simulink model "Curvature_lookup_table"  (R2021a)
settings: configuration reference "AION_IDS_Speedgoat" (kept outside this file)
libraries: simulink x1
settings Model: DataDictionary=Curvature_Lookup_Table.sldd  Creator=xinrui  LastModifiedBy=Administrator
settings ConfigSetRef: SourceName=AION_IDS_Speedgoat

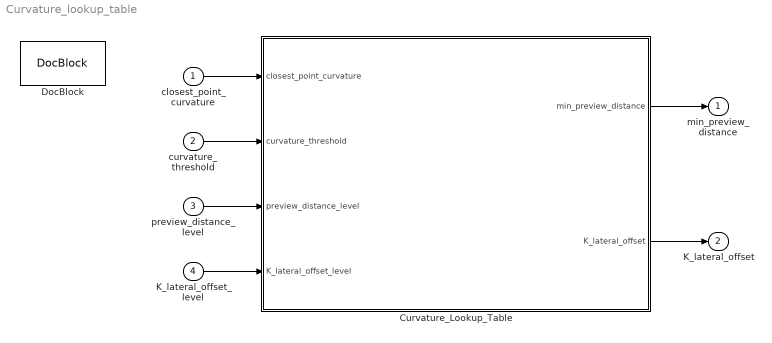
== system Curvature_lookup_table ==
  closest_point_curvature : Inport  OutDataTypeStr=double  PortDimensions=1
  curvature_threshold : Inport  Port=2  OutDataTypeStr=double  PortDimensions=6
  preview_distance_level : Inport  Port=3  OutDataTypeStr=double  PortDimensions=6
  K_lateral_offset_level : Inport  Port=4  OutDataTypeStr=double  PortDimensions=6
  Curvature_Lookup_Table : MATLAB Function  TreatAsAtomicUnit=on
  DocBlock : simulink/Model-Wide Utilities/DocBlock  DocumentType=HTML  mask(DocBlock){}
      mask Display:
      | plot([.8 0 0 1 1 .8 .8 1],[1 1 0 0 .8 1 .8 .8]);
      | text(.5,.6,'CHANGELOG','horizontalalignment','center');
      | text(.95,.05,get_param(gcb,'DocumentType'),'verticalalignment','bottom','horizontalalignment','right');
  min_preview_distance : Outport  OutDataTypeStr=double  PortDimensions=1
  K_lateral_offset : Outport  Port=2  OutDataTypeStr=double  PortDimensions=1
  wires:
  closest_point_curvature/1 -> Curvature_Lookup_Table/1(closest_point_curvature)
  curvature_threshold/1 -> Curvature_Lookup_Table/2(curvature_threshold)
  preview_distance_level/1 -> Curvature_Lookup_Table/3(preview_distance_level)
  K_lateral_offset_level/1 -> Curvature_Lookup_Table/4(K_lateral_offset_level)
  Curvature_Lookup_Table/1(min_preview_distance) -> min_preview_distance/1
  Curvature_Lookup_Table/2(K_lateral_offset) -> K_lateral_offset/1

== matlab function Curvature_lookup_table/Curvature_Lookup_Table ==
  data: closest_point_curvature input double size=1; curvature_threshold input double size=6; min_preview_distance output double size=1; K_lateral_offset output double size=1; preview_distance_level input double size=6; K_lateral_offset_level input double size=6
% 曲率查表
function [min_preview_distance, K_lateral_offset] = ...
    Curvature_lookup_table(closest_point_curvature, ...
    curvature_threshold, preview_distance_level, K_lateral_offset_level)
%   1.输入参数：
%       (1)closest_point_curvature              最近点曲率，1/m
%       (2)curvature_threshold                  曲率阈值，1/m
%       (3)preview_distance_level               预瞄距离等级，m
%       (4)K_lateral_offset_level               横向偏差矫正系数等级
%   2.输出参数：
%       (1)fixed_preview_distance               固定预瞄距离，m
%       (2)K_lateral_offset                     横向偏差矫正系数

%% 初始化
% 采用最大曲率阈值作为初始值，在曲率超过最大阈值时生效
min_preview_distance = preview_distance_level(end);
K_lateral_offset = K_lateral_offset_level(end);

%% 对最近点曲率绝对值查表确定其他输出数值
for index = 1 : 6
    if curvature_threshold(index) > abs(closest_point_curvature)
        min_preview_distance = preview_distance_level(index);
        K_lateral_offset = K_lateral_offset_level(index);
        break;
    end
end

end
